simulink model "RedCrane_kinematic_model_telescope"  (R2024a)
settings: Solver=FixedStepAuto  StartTime=0.0  StopTime=40  FixedStep=Ts  MaxStep=0.005  RelTol=1e-3
values from neighbouring files (symbols this model uses):
  Cartesian_home = [3.55, 0.4, 1.6]'    [enviroment_setup.m]
  telescope0 = 0    [enviroment_setup.m]
  thetaList0 = [0, 0,-pi/8, 0, 0]'    [enviroment_setup.m]
  Ts = 0.001    [enviroment_setup.m]
undefined symbols (not defined in the file or in its folder): dp_k_angle_to_stroke, dp_m_angle_to_stroke, p_k_angle_to_stroke, p_k_stroke_to_angle, p_m_angle_to_stroke, p_m_stroke_to_angle, X, Y, Z
libraries: sm_lib x82, nesl_utility x19, fl_lib x16
(part 1 of 3)
settings Model: Creator=sindr  LastModifiedBy=larso
settings RTWCC: GPUComputeCapability=3.5
settings ConfigComp: PLC_OutputDir=plc_export\FB_ForwardKinematicsTelescope  PLC_TargetIDE=twincat3  PLC_MultiTBSigbuilderTimeRange=off  PLC_FoldFBCallOutputVar=off  PLC_RemoveUnusedSSMethodCallArguments=off  PLC_UseCallOutputArgSyntax=off  PLC_EnableUnsignedAndDoubleTypes=off  PLC_EnableUDTSplitting=off  PLC_MaxFieldsInUDT=500  PLC_InlineEnumCastFunction=off

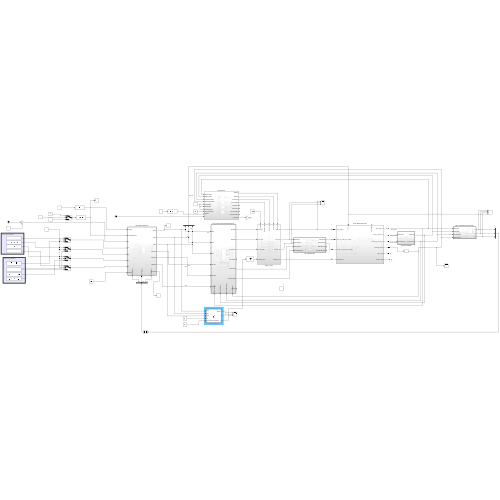
[thumbnail: Simulink's stored preview of the top-level diagram]
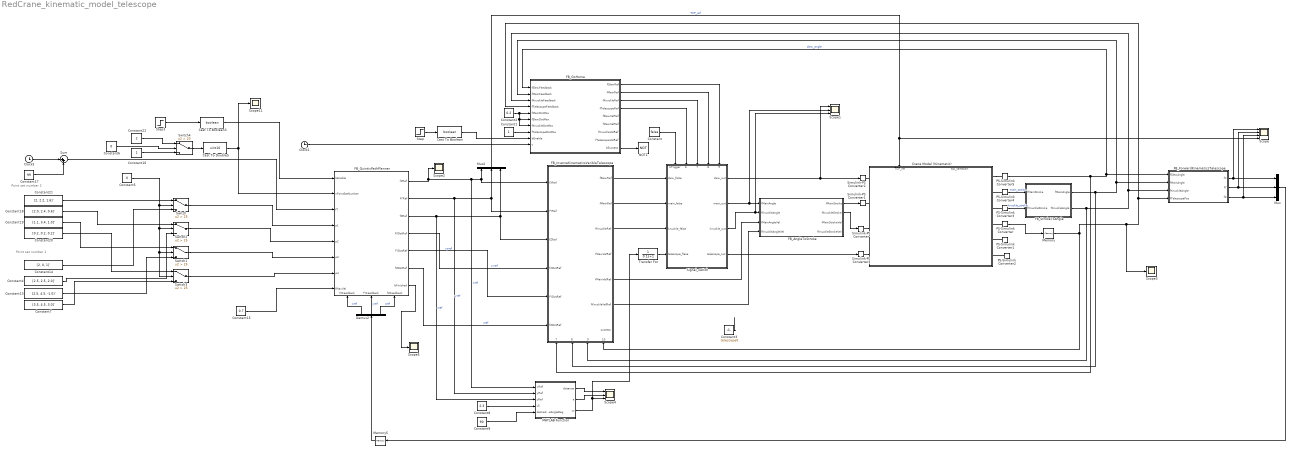
== system RedCrane_kinematic_model_telescope ==
  note: Point set number 2
  note: Point set number 1
  Cast To Boolean : DataTypeConversion  OutDataTypeStr=boolean  SaturateOnIntegerOverflow=off  RndMeth=Floor
  Cast To Boolean3 : DataTypeConversion  OutDataTypeStr=boolean  SaturateOnIntegerOverflow=off  RndMeth=Floor
  Cast To Double5 : DataTypeConversion  OutDataTypeStr=uint16  SaturateOnIntegerOverflow=off  RndMeth=Floor
  Clock1 : Clock
  Clock3 : Clock
  Constant : Constant  Value=false
  Constant1 : Constant
  Constant13 : Constant  Value=[2.5, 4.5, -1.0]'
  Constant14 : Constant  Value=[2, 0, 1]'
  Constant15 : Constant  Value=0.7
  Constant16 : Constant
  Constant17 : Constant  Value=99
  Constant18 : Constant  Value=[2.0, 2.4, 0.6]'
  Constant19 : Constant  Value=[1.1, 3.4, 1.0]'
  Constant2 : Constant  Value=0.2
  Constant20 : Constant  Value=[0.2, 0.2, 0.2]'
  Constant21 : Constant  Value=[2, 2.2, 1.6]'
  Constant22 : Constant  Value=2
  Constant3 : Constant  Value=telescope0
  Constant4 : Constant  Value=[2.5, 2.5, 2.0]'
  Constant5 : Constant  Value=0
  Constant6 : Constant  Value=0
  Constant7 : Constant  Value=[3.5, 4.5, 3.0]'
  Constant8 : Constant  Value=2.3
  Constant9 : Constant  Value=90
  Crane Model (Kinematic) : Subsystem
      settings: PortSchema="{\"entries\":[{\"content\":{\"sides\":[{\"content\":{\"connectorIds\":[\"LConn1\",\"LConn2\",\"LConn3\",\"LConn4\"]},\"type\":\"ConnectorPlacement.EquallySpacedRectSide\",\"uuid\":\"4a665765-5f1a-426d-91c2-f3af20fe3627\"},{\"content\":{\"connectorIds\":[\"RConn1\",\"RConn2\",\"RConn3\",\"RConn4\",\"RConn5\",\"RConn6\"],\"side\":\"RIGHT\"},\"type\":\"ConnectorPlacement.EquallySpacedRectSide\",\"uuid\":\"cf43645c-9a50-4bc9-b355-f38e72b1430d\"},{\"content\":{\"connectorIds\":[\"In1\",\"Out1\"],\"side\":\"TOP\"},\"type\":\"ConnectorPlacement.EquallySpacedRectSide\",\"uuid\":\"253dbb23-7a12-4bfe-bf07-7d8403188f09\"}]},\"type\":\"ConnectorPlacement.EquallySpacedConnector\",\"uuid\":\"5ffb1dcc-76b9-4b5c-ba8f-4653fe2f07c9\"}],\"packageUris\":[\"http://schema.mathworks.com/mf0/Connector/R2020b\"],\"version\":\"1.0\"}"
  Demux2 : Demux  Outputs=3
  FB_AngleToStroke : Subsystem  TreatAsAtomicUnit=on
  FB_ForwardKinematicsTelescope : Subsystem  TreatAsAtomicUnit=on
  FB_GoHome : Subsystem
  FB_InverceKinematicsVaribleTelescope : Subsystem  TreatAsAtomicUnit=on
      settings: PortSchema="{\"entries\":[{\"content\":{\"sides\":[{\"content\":{\"connectorIds\":[\"In1\",\"In2\",\"In3\",\"In4\",\"In5\",\"In6\"]},\"type\":\"ConnectorPlacement.EquallySpacedRectSide\",\"uuid\":\"b7f3f39a-cc1b-4519-b948-004466b4d293\"},{\"content\":{\"connectorIds\":[\"Out1\",\"Out2\",\"Out3\",\"Out4\",\"Out5\",\"Out6\",\"Out7\"],\"side\":\"RIGHT\"},\"type\":\"ConnectorPlacement.EquallySpacedRectSide\",\"uuid\":\"cf571c2f-2cc7-4d1d-bbc1-a75d80a0878e\"},{\"content\":{\"side\":\"TOP\"},\"type\":\"ConnectorPlacement.EquallySpacedRectSide\",\"uuid\":\"3f697bd9-7750-4474-8da5-1be48ba53c7e\"},{\"content\":{\"connectorIds\":[\"In7\",\"In8\",\"In9\",\"In10\"],\"side\":\"BOTTOM\"},\"type\":\"ConnectorPlacement.EquallySpacedRectSide\",\"uuid\":\"03fa0a4e-eedb-4a48-8076-446c86a2b4f7\"}]},\"type\":\"ConnectorPlacement.EquallySpacedConnector\",\"uuid\":\"6732c767-80e6-425f-b878-60bd961dd78b\"}],\"packageUris\":[\"http://schema.mathworks.com/mf0/Connector/R2020b\"],\"version\":\"1.0\"}"
  FB_QuinticPathPlanner : Subsystem  TreatAsAtomicUnit=on
      settings: PortSchema="{\"entries\":[{\"content\":{\"sides\":[{\"content\":{\"connectorIds\":[\"In1\",\"In2\",\"In3\",\"In4\",\"In5\",\"In6\",\"In7\",\"In8\"]},\"type\":\"ConnectorPlacement.EquallySpacedRectSide\",\"uuid\":\"4afc44f5-1297-406e-8d87-a7be537a6d64\"},{\"content\":{\"connectorIds\":[\"Out1\",\"Out2\",\"Out3\",\"Out4\",\"Out5\",\"Out6\",\"Out7\"],\"side\":\"RIGHT\"},\"type\":\"ConnectorPlacement.EquallySpacedRectSide\",\"uuid\":\"7afe290e-04ad-466c-95bd-018f979ae25c\"},{\"content\":{\"side\":\"TOP\"},\"type\":\"ConnectorPlacement.EquallySpacedRectSide\",\"uuid\":\"02dfa4f7-7b19-498a-9f4f-13236ded64ac\"},{\"content\":{\"connectorIds\":[\"In9\",\"In10\",\"In11\"],\"side\":\"BOTTOM\"},\"type\":\"ConnectorPlacement.EquallySpacedRectSide\",\"uuid\":\"8c67fe32-d6c8-4418-bdb4-feacce71c717\"}]},\"type\":\"ConnectorPlacement.EquallySpacedConnector\",\"uuid\":\"f03116da-160b-4aed-9148-ff690f14be69\"}],\"packageUris\":[\"http://schema.mathworks.com/mf0/Connector/R2020b\"],\"version\":\"1.0\"}"
  FB_StrokeToAngle : Subsystem  TreatAsAtomicUnit=on
  MATLAB Function : MATLAB Function  TreatAsAtomicUnit=on
  Memory : Memory  InitialCondition=telescope0
  Memory5 : Memory  InitialCondition=[Cartesian_home(1), Cartesian_home(2), Cartesian_home(3)]'
  Mux : Mux  Inputs=3
  Mux2 : Mux  Inputs=3
  NOT1 : Logic  Operator=NOT  IconShape=distinctive  AllPortsSameDT=off  OutDataTypeStr=boolean
  PS-Simulink Converter{,1..5} (6 alike) : nesl_utility/PS-Simulink Converter  PhysicalDomain=network_engine_domain  SubClassName=ps_output  LeftPortType=input  RightPortType=output  PseudoPeriodic=off  Frequencies=[]  VectorFormat=inherit  Unit=inherit  AffineConversion=off
  Scope : Scope  NumInputPorts=4
  Scope1 : Scope  NumInputPorts=3
  Scope{2..3,5,11} (4 alike) : Scope
  Scope4 : Scope  NumInputPorts=3
  Signal_switch : Subsystem
      settings: PortSchema="{\"entries\":[{\"content\":{\"sides\":[{\"content\":{\"connectorIds\":[\"In1\",\"In2\",\"In3\",\"In4\"]},\"type\":\"ConnectorPlacement.EquallySpacedRectSide\",\"uuid\":\"677999b9-dfe1-4592-affa-fb9b7d257ea0\"},{\"content\":{\"connectorIds\":[\"Out1\",\"Out2\",\"Out3\",\"Out4\"],\"side\":\"RIGHT\"},\"type\":\"ConnectorPlacement.EquallySpacedRectSide\",\"uuid\":\"3f36c443-9717-41bf-801d-3d95a9d66f59\"},{\"content\":{\"connectorIds\":[\"In5\",\"In6\",\"In7\",\"In8\",\"In9\"],\"side\":\"TOP\"},\"type\":\"ConnectorPlacement.EquallySpacedRectSide\",\"uuid\":\"b7ea9b48-8dcd-4abb-ae26-aa1832701a6a\"}]},\"type\":\"ConnectorPlacement.EquallySpacedConnector\",\"uuid\":\"7d55d43f-82cc-482c-a650-cc44ad6cee22\"}],\"packageUris\":[\"http://schema.mathworks.com/mf0/Connector/R2020b\"],\"version\":\"1.0\"}"
  Simulink-PS Converter{,1..3} (4 alike) : nesl_utility/Simulink-PS Converter  PhysicalDomain=network_engine_domain  SubClassName=ps_input  LeftPortType=input  RightPortType=output  PseudoPeriodic=off  Frequencies=[]  NoiseDistribution=none  NoiseParameters=[]  Unit=1  AffineConversion=off  FilteringAndDerivatives=filter  SimscapeFilterOrder=2  InputFilterTimeConstant=0.001  UdotUserProvided=0
  Step : Step  SampleTime=0
  Step3 : Step  Time=5  SampleTime=0
  Sum : Sum  Inputs=|++
  Switch{,1..3} (4 alike) : Switch  Criteria=u2 > Threshold  Threshold=25  SaturateOnIntegerOverflow=off  InputSameDT=off
  Switch4 : Switch  Criteria=u2 > Threshold  Threshold=20  SaturateOnIntegerOverflow=off  InputSameDT=off
  Transfer Fcn : TransferFcn  Denominator=[0.1 1]
  wires:
  FB_AngleToStroke/2(fKnuckleStroke) -> Simulink-PS Converter/1
  Mux2/1 -> Scope/4, Crane Model (Kinematic)/1(TCP_ref)  "TCP_ref"
  PS-Simulink Converter5/1 -> FB_ForwardKinematicsTelescope/1(fSlewAngle), FB_GoHome/1(fSlewFeedback), FB_InverceKinematicsVaribleTelescope/7(fSlewFeedback)  "slew_angle"
  Constant2/1 -> FB_GoHome/5(fMainDotMax), FB_GoHome/7(fKnuckleDotMax), FB_GoHome/6(fSlewDotMax)
  Cast To Boolean/1 -> FB_GoHome/9(bEnable)
  Step/1 -> Cast To Boolean/1
  FB_GoHome/9(bSuccess) -> NOT1/1
  Constant1/1 -> FB_GoHome/8(fTelescopeDotMax)
  Clock1/1 -> FB_GoHome/10(t)
  FB_StrokeToAngle/2(fKnuckleAngle) -> FB_GoHome/3(fKnuckleFeedback), FB_ForwardKinematicsTelescope/3(fKnuckleAngle), FB_InverceKinematicsVaribleTelescope/9(fKnuckleFeedback)
  FB_StrokeToAngle/1(fMainAngle) -> FB_GoHome/2(fMainFeedback), FB_ForwardKinematicsTelescope/2(fMainAngle), FB_InverceKinematicsVaribleTelescope/8(fMainFeedback)
  PS-Simulink Converter4/1 -> FB_StrokeToAngle/1(fMainStroke)  "main_stroke"
  PS-Simulink Converter3/1 -> FB_StrokeToAngle/2(fKnuckleStroke)  "knuckle_stroke"
  FB_InverceKinematicsVaribleTelescope/5(fMainVelRef) -> FB_AngleToStroke/3(fMainAngleVel)
  FB_InverceKinematicsVaribleTelescope/6(fKnuckleVelRef) -> FB_AngleToStroke/4(fKnuckleAngleVel)
  FB_GoHome/1(fSlewRef) -> Signal_switch/9(slew_true)
  FB_GoHome/2(fMainRef) -> Signal_switch/8(main_true)
  FB_GoHome/3(fKnuckleRef) -> Signal_switch/7(knuckle_true)
  FB_GoHome/4(fTelescopeRef) -> Signal_switch/6(telescope_true)
  Constant/1 -> Signal_switch/5(bTrigger)
  FB_InverceKinematicsVaribleTelescope/1(fSlewRef) -> Signal_switch/1(slew_false)
  FB_InverceKinematicsVaribleTelescope/2(fMainRef) -> Signal_switch/2(main_false)
  FB_InverceKinematicsVaribleTelescope/3(fKnuckleRef) -> Signal_switch/3(knuckle_false)
  Signal_switch/1(slew_out) -> Scope1/1, Simulink-PS Converter2/1
  Signal_switch/2(main_out) -> Scope1/2, FB_AngleToStroke/1(fMainAngle)
  Signal_switch/3(knuckle_out) -> Scope1/3, FB_AngleToStroke/2(fKnuckleAngle)
  FB_AngleToStroke/1(fMainStroke) -> Simulink-PS Converter1/1
  FB_QuinticPathPlanner/1(fXRef) -> Scope2/1, MATLAB Function/1(xRef), FB_InverceKinematicsVaribleTelescope/1(fXRef), Mux2/1  "xref"
  FB_QuinticPathPlanner/2(fYRef) -> MATLAB Function/2(yRef), Mux2/2, FB_InverceKinematicsVaribleTelescope/2(fYRef)  "yref"
  FB_QuinticPathPlanner/3(fZRef) -> MATLAB Function/3(zRef), Mux2/3, FB_InverceKinematicsVaribleTelescope/3(fZRef)  "zref"
  FB_QuinticPathPlanner/4(fXDotRef) -> FB_InverceKinematicsVaribleTelescope/4(fXDotRef)  "vxref"
  FB_QuinticPathPlanner/5(fYDotRef) -> FB_InverceKinematicsVaribleTelescope/5(fYDotRef)  "vyref"
  FB_ForwardKinematicsTelescope/1(fX) -> Scope/1, Mux/1
  FB_ForwardKinematicsTelescope/2(fY) -> Scope/2, Mux/2
  FB_ForwardKinematicsTelescope/3(fZ) -> Scope/3, Mux/3
  Constant14/1 -> Switch/3
  Switch2/1 -> FB_QuinticPathPlanner/5(p2)
  Switch3/1 -> FB_QuinticPathPlanner/7(p4)
  Switch1/1 -> FB_QuinticPathPlanner/6(p3)
  Switch/1 -> FB_QuinticPathPlanner/4(p1)
  Cast To Boolean3/1 -> FB_QuinticPathPlanner/1(bEnable)
  Sum/1 -> FB_QuinticPathPlanner/3(fT)
  Step3/1 -> Cast To Boolean3/1
  Constant21/1 -> Switch/1
  Mux/1 -> Memory5/1
  Constant18/1 -> Switch2/1
  Switch4/1 -> Cast To Double5/1
  Constant22/1 -> Switch4/1
  Cast To Double5/1 -> FB_QuinticPathPlanner/2(nPointSetNumber), Scope11/1
  Constant16/1 -> Switch4/3
  Constant20/1 -> Switch3/1
  Constant13/1 -> Switch1/3
  Constant7/1 -> Switch3/3
  Constant4/1 -> Switch2/3
  Constant15/1 -> FB_QuinticPathPlanner/8(fMaxVel)
  Clock3/1 -> Sum/1
  Constant19/1 -> Switch1/1
  Constant17/1 -> Sum/2
  FB_QuinticPathPlanner/6(fZDotRef) -> FB_InverceKinematicsVaribleTelescope/6(fZDotRef)  "zref"
  Memory5/1 -> Demux2/1
  Demux2/1 -> FB_QuinticPathPlanner/9(fXFeedback)  "xref"
  Demux2/2 -> FB_QuinticPathPlanner/10(fYFeedback)  "yref"
  Demux2/3 -> FB_QuinticPathPlanner/11(fZFeedback)  "zref"
  Constant5/1 -> Switch3/2, Switch1/2, Switch2/2, Switch/2
  Constant6/1 -> Switch4/2
  Signal_switch/4(telescope_out) -> Simulink-PS Converter3/1
  PS-Simulink Converter/1 -> Memory/1
  MATLAB Function/1(distance) -> Scope4/1
  MATLAB Function/2(a) -> Scope4/2
  MATLAB Function/3(xt) -> Transfer Fcn/1, Scope4/3
  Memory/1 -> FB_ForwardKinematicsTelescope/4(fTelescopePos), FB_GoHome/4(fTelescopeFeedback), Scope3/1, FB_InverceKinematicsVaribleTelescope/10(fTelescopePos)
  Transfer Fcn/1 -> Signal_switch/4(telescope_flase)
  Constant3/1 -> ?
  FB_QuinticPathPlanner/7(bFinished) -> Scope5/1
  Constant8/1 -> MATLAB Function/4(L5)
  Constant9/1 -> MATLAB Function/5(desiredKnuckleAngleDeg)
  connections:
  Simulink-PS Converter/RConn1 -- Crane Model (Kinematic)/LConn3
  Simulink-PS Converter2/RConn1 -- Crane Model (Kinematic)/LConn1
  Simulink-PS Converter1/RConn1 -- Crane Model (Kinematic)/LConn2
  Simulink-PS Converter3/RConn1 -- Crane Model (Kinematic)/LConn4
  PS-Simulink Converter/LConn1 -- Crane Model (Kinematic)/RConn4
  PS-Simulink Converter1/LConn1 -- Crane Model (Kinematic)/RConn5
  PS-Simulink Converter2/LConn1 -- Crane Model (Kinematic)/RConn6
  PS-Simulink Converter3/LConn1 -- Crane Model (Kinematic)/RConn3
  PS-Simulink Converter4/LConn1 -- Crane Model (Kinematic)/RConn2
  Crane Model (Kinematic)/RConn1 -- PS-Simulink Converter5/LConn1
